simulink model "lab1_ErrorSpace_Approach"  (R2020b)
settings: Solver=VariableStepAuto  StartTime=0.0  StopTime=10.0  RelTol=1e-3
undefined symbols (not defined in the file): A_r, A_r1, A_r2, D_H_s, D_w, degs2rpm, enable_Reference, K_eps, N_H_s, N_w, rpm2rads, sens, w_0, w_1
settings Model: Creator=Musta  LastModifiedBy=Musta

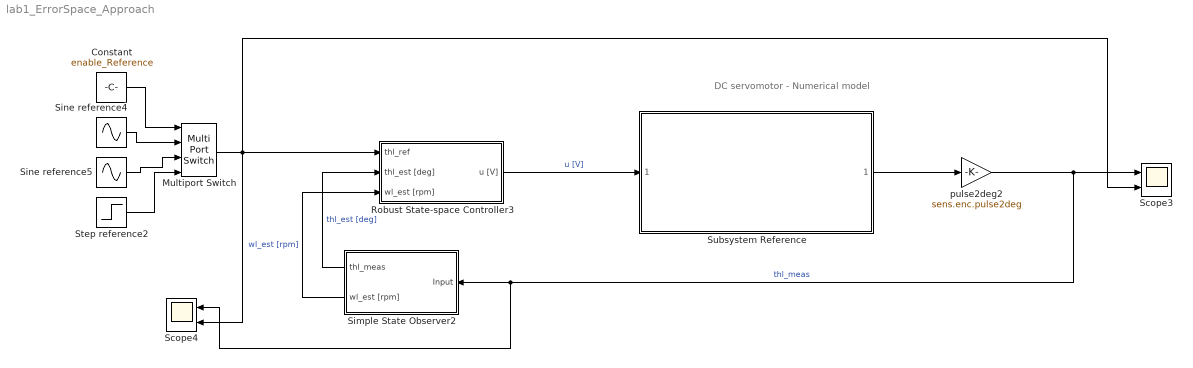
== system lab1_ErrorSpace_Approach ==
  note: DC servomotor - Numerical model
  Constant : Constant  Value=enable_Reference
  Multiport Switch : MultiPortSwitch
  Robust State-space Controller3 : Subsystem
  Scope3 : Scope  NumInputPorts=2
  Scope4 : Scope  NumInputPorts=2
  Simple State Observer2 : Subsystem
  Sine reference4 : Sin  Amplitude=A_r  Frequency=w_0  SampleTime=0
  Sine reference5 : Sin  Amplitude=A_r1  Frequency=w_1  SampleTime=0
  Step reference2 : Step  Time=0  After=A_r2  SampleTime=0
  Subsystem Reference : Subsystem  ReferencedSubsystem=plant_Model
  pulse2deg2 : Gain  Gain=sens.enc.pulse2deg
  wires:
  Robust State-space Controller3/1(u [V]) -> Subsystem Reference/1  "u [V]"
  Simple State Observer2/2(wl_est [rpm]) -> Robust State-space Controller3/3(wl_est [rpm])  "wl_est [rpm]"
  Simple State Observer2/1(thl_meas) -> Robust State-space Controller3/2(thl_est [deg])  "thl_est [deg]"
  Multiport Switch/1 -> Scope4/2, Robust State-space Controller3/1(thl_ref), Scope3/2
  Sine reference4/1 -> Multiport Switch/2
  Sine reference5/1 -> Multiport Switch/3
  Subsystem Reference/1 -> pulse2deg2/1
  pulse2deg2/1 -> Scope4/1, Simple State Observer2/1(Input), Scope3/1  "thl_meas"
  Constant/1 -> Multiport Switch/1
  Step reference2/1 -> Multiport Switch/4

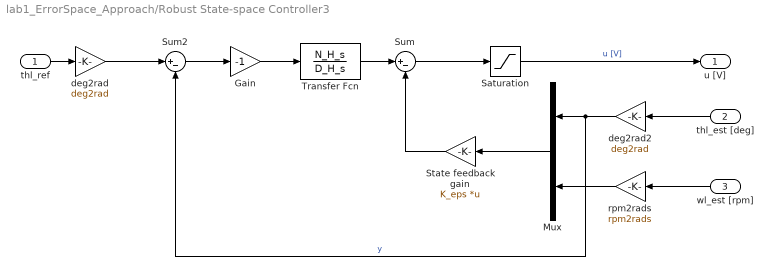
== system lab1_ErrorSpace_Approach/Robust State-space Controller3 ==
  thl_ref : Inport
  thl_est [deg] : Inport  Port=2
  wl_est [rpm] : Inport  Port=3
  Gain : Gain  Gain=-1
  Mux : Mux  Inputs=2
  Saturation : Saturate  UpperLimit=10  LowerLimit=-10
  State feedback gain : Gain  Gain=K_eps  Multiplication=Matrix(K*u)
  Sum : Sum  Inputs=|+-
  Sum2 : Sum  Inputs=|+-
  Transfer Fcn : TransferFcn  Numerator=N_H_s  Denominator=D_H_s
  deg2rad : Gain  Gain=deg2rad
  deg2rad2 : Gain  Gain=deg2rad
  rpm2rads : Gain  Gain=rpm2rads
  u [V] : Outport
  wires:
  Mux/1 -> State feedback gain/1
  deg2rad/1 -> Sum2/1
  thl_ref/1 -> deg2rad/1
  Saturation/1 -> u [V]/1  "u [V]"
  rpm2rads/1 -> Mux/2
  wl_est [rpm]/1 -> rpm2rads/1
  thl_est [deg]/1 -> deg2rad2/1
  deg2rad2/1 -> Sum2/2, Mux/1  "y"
  Sum/1 -> Saturation/1
  Sum2/1 -> Gain/1
  Transfer Fcn/1 -> Sum/1
  State feedback gain/1 -> Sum/2
  Gain/1 -> Transfer Fcn/1

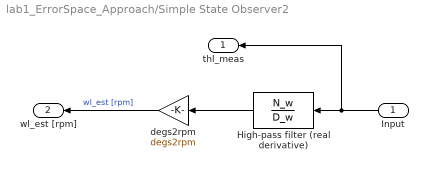
== system lab1_ErrorSpace_Approach/Simple State Observer2 ==
  Input : Inport
  High-pass filter (real derivative) : TransferFcn  Numerator=N_w  Denominator=D_w
  degs2rpm : Gain  Gain=degs2rpm
  thl_meas : Outport
  wl_est [rpm] : Outport  Port=2
  wires:
  Input/1 -> thl_meas/1, High-pass filter (real derivative)/1
  High-pass filter (real derivative)/1 -> degs2rpm/1
  degs2rpm/1 -> wl_est [rpm]/1  "wl_est [rpm]"
